simulink model "ODE_Fucn2"  (R2020a)
settings: Solver=VariableStepAuto  StartTime=0.0  StopTime=10.0  RelTol=1e-3
values from neighbouring files (symbols this model uses):
  A = [ 0 1; -1 -2]    [my_main.m]
  B = [ 0; 1]    [my_main.m]
  beta_gain = 1    [my_main.m]
  c = 1    [my_main.m]
  ini = [2;2]    [my_main.m]
  k = 1    [my_main.m]
settings Model: Creator=TA  LastModifiedBy=TA

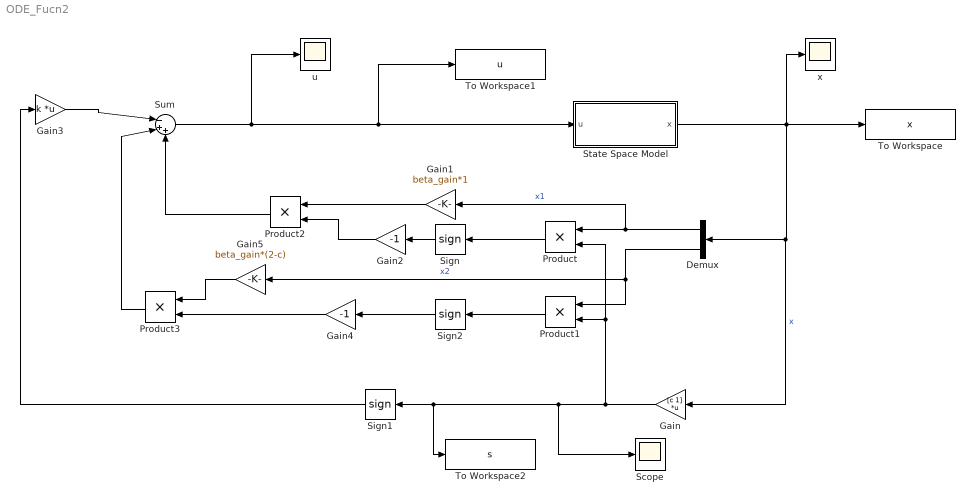
== system ODE_Fucn2 ==
  Demux : Demux  Outputs=2
  Gain : Gain  Gain=[c 1]  Multiplication=Matrix(K*u) (u vector)
  Gain1 : Gain  Gain=beta_gain*1
  Gain2 : Gain  Gain=-1
  Gain3 : Gain  Gain=k  Multiplication=Matrix(K*u) (u vector)
  Gain4 : Gain  Gain=-1
  Gain5 : Gain  Gain=beta_gain*(2-c)
  Product{,1..3} (4 alike) : Product
  Scope : Scope
  Sign : Signum
  Sign1 : Signum
  Sign2 : Signum
  State Space Model : Subsystem
  Sum : Sum  Inputs=|-++
  To Workspace : ToWorkspace  VariableName=x  SampleTime=-1
  To Workspace1 : ToWorkspace  VariableName=u  SaveFormat=Timeseries  SampleTime=-1
  To Workspace2 : ToWorkspace  VariableName=s  SaveFormat=Timeseries  SampleTime=-1
  u : Scope
  x : Scope
  wires:
  State Space Model/1(x) -> Gain/1, Demux/1, x/1, To Workspace/1  "x"
  Demux/1 -> Gain1/1, Product/1  "x1"
  Demux/2 -> Gain5/1, Product1/1  "x2"
  Gain/1 -> Scope/1, To Workspace2/1, Sign1/1, Product/2, Product1/2
  Gain1/1 -> Product2/1
  Product/1 -> Sign/1
  Sign/1 -> Gain2/1
  Gain2/1 -> Product2/2
  Sum/1 -> u/1, To Workspace1/1, State Space Model/1(u)
  Product2/1 -> Sum/3
  Sign1/1 -> Gain3/1
  Gain3/1 -> Sum/1
  Product1/1 -> Sign2/1
  Sign2/1 -> Gain4/1
  Gain5/1 -> Product3/1
  Gain4/1 -> Product3/2
  Product3/1 -> Sum/2

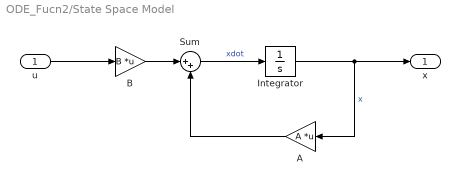
== system ODE_Fucn2/State Space Model ==
  u : Inport
  A : Gain  Gain=A  Multiplication=Matrix(K*u) (u vector)
  B : Gain  Gain=B  Multiplication=Matrix(K*u) (u vector)
  Integrator : Integrator  InitialCondition=ini
  Sum : Sum  Inputs=|++
  x : Outport
  wires:
  u/1 -> B/1
  B/1 -> Sum/1
  Sum/1 -> Integrator/1  "xdot"
  Integrator/1 -> A/1, x/1  "x"
  A/1 -> Sum/2
